simulink model "Testing_Kin"  (R2017b)
settings: Solver=VariableStepAuto  StartTime=0.0  StopTime=10.0  RelTol=1e-3
InitFcn:
  | l1 = 0.475;
  | l2 = 0.465;
  | l3 = 0.62;
  | h = 0.3;
  | limit_linear_P = 0.75;
  | limit_linear_N = -0.75;
settings Model: Creator=aiellog  LastModifiedBy=aiellog

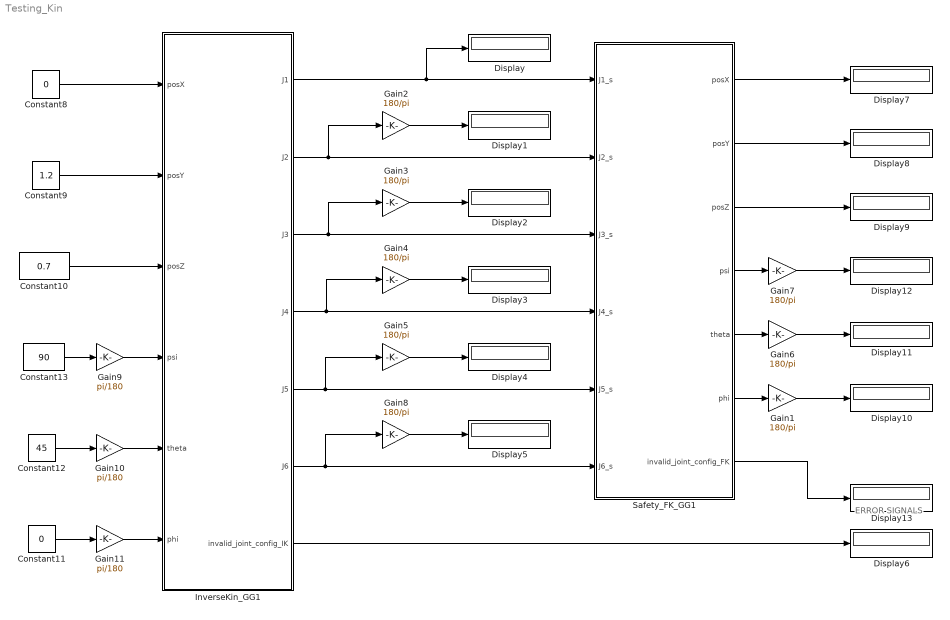
== system Testing_Kin ==
  note: ERROR SIGNALS
  Constant10 : Constant  Value=0.7  OutDataTypeStr=double
  Constant11 : Constant  Value=0  OutDataTypeStr=double
  Constant12 : Constant  Value=45  OutDataTypeStr=double
  Constant13 : Constant  Value=90  OutDataTypeStr=double
  Constant8 : Constant  Value=0  OutDataTypeStr=double
  Constant9 : Constant  Value=1.2  OutDataTypeStr=double
  Display{,1..13} (14 alike) : Display
  Gain{1..8} (8 alike) : Gain  Gain=180/pi
  Gain10 : Gain  Gain=pi/180
  Gain11 : Gain  Gain=pi/180
  Gain9 : Gain  Gain=pi/180
  InverseKin_GG1 : MATLAB Function  TreatAsAtomicUnit=on
  Safety_FK_GG1 : MATLAB Function  TreatAsAtomicUnit=on
  wires:
  InverseKin_GG1/4(J4) -> Gain4/1, Safety_FK_GG1/4(J4_s)
  InverseKin_GG1/3(J3) -> Gain3/1, Safety_FK_GG1/3(J3_s)
  Gain5/1 -> Display4/1
  Constant9/1 -> InverseKin_GG1/2(posY)
  Constant13/1 -> Gain9/1
  Constant12/1 -> Gain10/1
  Constant10/1 -> InverseKin_GG1/3(posZ)
  InverseKin_GG1/2(J2) -> Gain2/1, Safety_FK_GG1/2(J2_s)
  Constant11/1 -> Gain11/1
  InverseKin_GG1/7(invalid_joint_config_IK) -> Display6/1
  Constant8/1 -> InverseKin_GG1/1(posX)
  Safety_FK_GG1/2(posY) -> Display8/1
  Safety_FK_GG1/4(psi) -> Gain7/1
  Safety_FK_GG1/6(phi) -> Gain1/1
  InverseKin_GG1/5(J5) -> Gain5/1, Safety_FK_GG1/5(J5_s)
  Gain4/1 -> Display3/1
  Safety_FK_GG1/7(invalid_joint_config_FK) -> Display13/1
  Gain3/1 -> Display2/1
  InverseKin_GG1/1(J1) -> Display/1, Safety_FK_GG1/1(J1_s)
  Gain2/1 -> Display1/1
  Safety_FK_GG1/3(posZ) -> Display9/1
  Safety_FK_GG1/5(theta) -> Gain6/1
  Safety_FK_GG1/1(posX) -> Display7/1
  Gain1/1 -> Display10/1
  Gain6/1 -> Display11/1
  Gain7/1 -> Display12/1
  InverseKin_GG1/6(J6) -> Gain8/1, Safety_FK_GG1/6(J6_s)
  Gain8/1 -> Display5/1
  Gain9/1 -> InverseKin_GG1/4(psi)
  Gain10/1 -> InverseKin_GG1/5(theta)
  Gain11/1 -> InverseKin_GG1/6(phi)

== matlab function Testing_Kin/InverseKin_GG1 ==
  data: J1 output; posX input; J2 output; J3 output; J4 output; J5 output; J6 output; posY input; posZ input; psi input; theta input; phi input; invalid_joint_config_IK output; l1 parameter; l2 parameter; l3 parameter; h parameter; limit_linear_P parameter; limit_linear_N parameter
function [J1,J2,J3,J4,J5,J6,invalid_joint_config_IK] = fcn(posX,posY,posZ,psi,theta,phi, l1, l2, l3, h, limit_linear_P, limit_linear_N)

% This function takes the 6 cartesian coordinates and returns the joint coordinates. 
% Naming:
%       posX: end effector x with respect to the base coordinates system
%       posY: end effector y with respect to the base coordinates system
%       posZ: end effector z with respect to the base coordinates system
%       psi: end effector Yaw angle 
%       theta: end effector Pitch angle 
%       phi: end effector Roll angle
%       J1: prismatic joint
%       J2: first rotational joint (around z axis)
%       J3: second rotational joint (coplanar with J4 and J5)
%       J4: third rotational joint (coplanar with J3 and J5)
%       J5: fourth rotational joint (coplanar with J3 and J4)
%       J6: fifth rotational joint (roll motion)

% Author: Aiello Gregorio, Gabor Kosa
% BIROMED Lab, University of Basel, 2017.

% Self collision IK, c4 > 1

invalid_joint_config_IK = 0; % this is the error signal for the inverse kinematics, initially set  to 0

if(posZ < -h) % the end effector cannot go under the table 
    posZ = -h;
    invalid_joint_config_IK = 1;
end

if(posY < 0) % the end effector cannot go behind the table 
    posY = 0;
    invalid_joint_config_IK = 1;
end


if(psi<0.0321) %robot cannot be parallel to the rail and can not turn backward
    psi=0.0321;
    invalid_joint_config_IK = 1;
elseif(psi > pi-(0.0321))
    psi=pi-(0.0321);
    invalid_joint_config_IK = 1;    
end

J1 = posX - posY/tan(psi); % Prismatic joint, DIV BY 0 CHECKED
if abs(J1) < 0.000001
    J1=0;
end

if(J1<-1.5 || J1 > 1.5)
    invalid_joint_config_IK = 1;
end

posR = sqrt((J1 - posX)^2 + posY^2); %distance of robot tip on plane of operation

J2 = psi; % First rotational joint controls the yaw rotation of the end effector
if abs(J2) < 0.000001
    J2=0;
end
J6 = phi; % Last rotatinal joint controls the roll rotation of the end effecotr
if abs(J6) < 0.000001
    J6=0;
end
Lrz = sqrt(posR^2+posZ^2); %check if length required from the robot in the operation plane exceeds l1+l2+l3

if(Lrz > (l1+l2+l3))
    posZ = (l1+l2+l3-.001)*sin(theta);
    posR = (l1+l2+l3-.001)*cos(theta);
    invalid_joint_config_IK = 1;
end
%if yes the robot is set to the boundary of the workspace


% J4 -------------------------

%1 is the position of joint J5 
lR = posR - l3*cos(theta);

lZ = posZ - l3*sin(theta);
if(lZ < -h)
   lZ = -h;
   invalid_joint_config_IK = 1;
end

lL = sqrt(lR*lR + lZ*lZ);
alpha = atan2(lZ, lR); %The angle of J5 on the operation plane, DIV BY 0


c4 = (- lL^2 + l1^2 + l2^2)/(2*l1*l2); % DIV BY 0 CHECKED

if c4 == 0 %avoid division by 0
    c4=1; % this is  a random value just used to not drive twincat crazy
    invalid_joint_config_IK = 1;
end

if(c4>0.9851) %the robots needs to get to a position that is over its ability in the R-Z plane
    c4 = 0.9851;
    invalid_joint_config_IK = 1;
elseif(c4 < -1) % self collision control
    c4 = -1;
    invalid_joint_config_IK = 1;
end
s4 = sqrt(1 - c4^2); %This angle can be only between 0 and pi therefore s4 between 0 and 1
J4 = - pi + atan2(s4,c4); % DIV BY 0 CHECKED

if(J4>pi) %J4 defined between -pi and pi
    J4 = J4 - 2*pi;
elseif(J4<-pi)
    J4 = J4 + 2*pi;
end
if abs(J4) < 0.000001
    J4=0;
end
% J3 -------------------------
c_beta = (-l2^2 + l1^2 + lL^2)/(2*l1*lL); % DIV BY 0 CHECKED
if(c_beta == 0)
    c_beta = 1; % this is  a random value just used to not drive twincat crazy
    invalid_joint_config_IK = 1;
end
if(c_beta>1)
    c_beta = 1;
    invalid_joint_config_IK = 1;
elseif(c_beta<-1)
    c_beta=-1;
    invalid_joint_config_IK = 1;    
end
s_beta = +sqrt(1 - c_beta^2);
beta = atan2(s_beta, c_beta); %The J5J3J4, % DIV BY 0 CHECKED
J3 = -(pi/2 - (alpha + beta));

if(J3>pi) %J3 defined between -pi and pi
    J3 = J3 - 2*pi;
elseif(J3<-pi)
    J3 = J3 + 2*pi;
end
if abs(J3) < 0.000001
    J3=0;
end
%-------------------------------------------------%
J5 = theta - J3 - J4 - pi/2;

if(J5>pi) %J5 defined between -pi and pi
    J5 = J5 - 2*pi;
elseif(J5<-pi)
    J5 = J5 + 2*pi;
if abs(J5) < 0.000001
    J5=0;
end

% Joint limitation and self collision avoidance---------------------------------
limit_linear_P = 0.75;
limit_linear_N = -0.75;

beta = pi+J4;
c = sqrt(l1^2+l2^2 - 2*l1*l2*cos(beta));
if c == 0 % avoid division by zero and return error
    c = 1; % this is  a random value just used to not drive twincat crazy
    invalid_joint_config_IK=1;
end
alpha = asin((l1*sin(beta))/c); % DIV BY 0 CHECKED

J3_max = asin(h/l1) + pi/2;

if J5 < -pi+alpha 
    invalid_joint_config_IK=1;
    J5 = -pi+alpha;
elseif J5 > pi*3/4 
    invalid_joint_config_IK=1;
    J5 = pi*3/4;
elseif J2 < 0 
    invalid_joint_config_IK=1;
    J2 = 0;
elseif J2 > pi
    invalid_joint_config_IK=1;
    J2 = pi;
elseif J4 > 0 
    invalid_joint_config_IK=1;
    J4 = 0;
elseif J4 < -pi 
    invalid_joint_config_IK=1;
    J4 = -pi;    
elseif J1 < limit_linear_N 
    invalid_joint_config_IK=1;
    J1 = limit_linear_N;        
elseif J1 > limit_linear_P 
    invalid_joint_config_IK=1;
    J1 = limit_linear_P;   
elseif J3 < -J3_max 
    invalid_joint_config_IK=1;
    J3 = -J3_max; 
elseif J3 > pi/2
    invalid_joint_config_IK=1;
    J3 = pi/2;     
elseif J6 < -pi 
    invalid_joint_config_IK=1;
    J6 = -pi ; 
elseif J6 > pi
    invalid_joint_config_IK=1;
    J6 = pi;
end

end

== matlab function Testing_Kin/Safety_FK_GG1 ==
  data: J1_s input; posX output; J2_s input; J3_s input; J4_s input; J5_s input; J6_s input; posY output; posZ output; psi output; theta output; phi output; invalid_joint_config_FK output; l1 parameter; l2 parameter; l3 parameter; h parameter; limit_linear_N parameter; limit_linear_P parameter
function [posX,posY,posZ,psi,theta,phi,invalid_joint_config_FK] = fcn(J1_s,J2_s,J3_s,J4_s,J5_s,J6_s, l1, l2, l3, h, limit_linear_N, limit_linear_P)

% This function takes the 6 joints variables and returns the end effector
% positions and orientation in cartesian coordinates. 
% Naming:
%       J1: prismatic joint
%       J2: first rotational joint (around z axis)
%       J3: second rotational joint (coplanar with J4 and J5)
%       J4: third rotational joint (coplanar with J3 and J5)
%       J5: fourth rotational joint (coplanar with J3 and J4)
%       J6: fifth rotational joint (roll motion)
%       posX: end effector x with respect to the base coordinates system
%       posY: end effector y with respect to the base coordinates system
%       posZ: end effector z with respect to the base coordinates system
%       psi: end effector Yaw angle 
%       theta: end effector Pitch angle 
%       phi: end effector Roll angle

% Author: Aiello Gregorio, Gabor Kosa
% BIROMED Lab, University of Basel, 2017.

invalid_joint_config_FK=0; % this is the error signal for the forward kinematics, initially set  to 0

J3_max = asin(h/l1) + pi/2; % maximum value for J3, (the zero is the vertical configuration)

%% ~~~~~~~~~~~~~~~~~~~~~~~~~~~~~~~~~~~~~~~~~~~~~~~~~~~~~~~~~~~~~~~~~~~~~~~~~%
% Boundaries
beta = pi+J4_s;
c = sqrt(l1^2+l2^2 - 2*l1*l2*cos(beta));
if c == 0 % avoid division by zero and return error
    c = 1; % this is  a random value just used to not drive twincat crazy
    invalid_joint_config_FK=1;
end
alpha = asin((l1*sin(beta))/c); % DIV BY 0 CHECKED
%~~~~~~~~~~~~~~~~~~~~~~~~~~~~~~~~~~~~~~~~~~~~~~~~~~~~~~~~~~~~~~~~~~~~~~~~~%

% Check for joint limits and illegal configuration
if J5_s < -pi+alpha 
    invalid_joint_config_FK=1;
    J5_s = -pi+alpha;
elseif J5_s > pi*3/4 
    invalid_joint_config_FK=1;
    J5_s = pi*3/4;
elseif J2_s < 0 
    invalid_joint_config_FK=1;
    J2_s = 0;
elseif J2_s > pi
    invalid_joint_config_FK=1;
    J2_s = pi;
elseif J4_s > 0 
    invalid_joint_config_FK=1;
    J4_s = 0;
elseif J4_s < -pi 
    invalid_joint_config_FK=1;
    J4_s = -pi;    
elseif J1_s < limit_linear_N 
    invalid_joint_config_FK=1;
    J1_s = limit_linear_N;        
elseif J1_s > limit_linear_P 
    invalid_joint_config_FK=1;
    J1_s = limit_linear_P;   
elseif J3_s < -J3_max 
    invalid_joint_config_FK=1;
    J3_s = -J3_max; 
elseif J3_s > pi/2
    invalid_joint_config_FK=1;
    J3_s = pi/2;     
elseif J6_s < -pi 
    invalid_joint_config_FK=1;
    J6_s = -pi ; 
elseif J6_s > pi
    invalid_joint_config_FK=1;
    J6_s = pi;
end

%% ~~~~~~~~~~~~~~~~~~~~~~~~~~~~~~~~~~~~~~~~~~~~~~~~~~~~~~~~~~~~~~~~~~~~~~~~ %
% Yaw angle
psi = J2_s;
if abs(psi) < 0.000001 % avoid useless precision
    psi=0;
end

%% ~~~~~~~~~~~~~~~~~~~~~~~~~~~~~~~~~~~~~~~~~~~~~~~~~~~~~~~~~~~~~~~~~~~~~~~~ %
% Roll angle
phi = J6_s; 
if abs(phi) < 0.000001 % avoid useless precision
    phi=0;
end

%% ~~~~~~~~~~~~~~~~~~~~~~~~~~~~~~~~~~~~~~~~~~~~~~~~~~~~~~~~~~~~~~~~~~~~~~~~ %
% Pitch angle
theta = + J3_s + J4_s + J5_s + pi/2;
if(theta > pi)
    theta = theta - 2*pi;
elseif(theta < -pi)
    theta = theta + 2*pi;
end

if abs(theta) < 0.000001 % avoid useless precision
    theta=0;
end


% Projection of the 3 aligned joints on the radial plane

xy_radial_length = (l1*sin(-J3_s) + l2*sin(-J3_s-J4_s) + l3*sin(-J3_s-J4_s-J5_s));
posX = J1_s + xy_radial_length*cos(J2_s);

if posX < 0.000001 % avoid useless precision
    posX=0;
end

posY = xy_radial_length*sin(J2_s);
if posY < 0
    invalid_joint_config_FK=1;
end

if abs(posY) < 0.000001 % avoid useless precision
    posY=0;
end

z_radial_length = l1*cos(-J3_s) + l2*cos(-J3_s-J4_s) + l3*cos(-J3_s-J4_s-J5_s);
posZ = z_radial_length;

if posZ < - h
    invalid_joint_config_FK=1;
end

if abs(posZ) < 0.000001 % avoid useless precision
    posZ=0;
end
